simulink model "alimentatorer"  (Simulink 10.0)
settings: Solver=ode15s  StartTime=0.0  StopTime=.5  FixedStep=1e-4  MaxStep=1e-3  RelTol=1e-6  AbsTol=1e-6  EnableMultiTasking=on
settings Model: Creator=prof. G. Celentano  LastModifiedBy=giuseppericcio  ExtModeTrigMode=oneshot  ExtModeArmWhenConnect=off
settings Model: LogicAnalyzerGraphicalSettings=|
  | {
  |   "cursors" : {
  |     "activeCursor" : 0,
  |     "lockedCursors" : [
  | 
  |     ],
  |     "startingCursor" : 0,
  |     "times" : [
  |       0.006
  |     ]
  |   },
  |   "global" : {
  |   },
  |   "panels" : [
  |     {
  |       "height" : 100,
  |       "startingTrace" : 0,
  |       "traces" : [
  | 
  |       ],
  |       "yOffset" : 0
  |     }
  |   ],
  |   "timeAxis" : {
  |     "pixelsPerSecond" : 104998.22050048786
  |   },
  |   "trigger" : {
  |     "enabled" : false,
  |     "mode" : "once",
  |     "samples" : 200,
  |     "signals" : {
  |     },
  |     "stages" : [
  |       {
  |         "conditions" : [
  | 
  |         ],
  |         "operator" : "AND"
  |       }
  |     ]
  |   }
  | }
settings SolverCC: AutoScaleAbsTol=off
settings DataIOCC: SignalLoggingName=sigsOut
settings OptimizationCC: BooleanDataType=off  ExpressionDepthLimit=2147483647
settings DebuggingCC: SaveWithParameterizedLinksMsg=none  SignalResolutionControl=TryResolveAllWithWarning  MultiTaskDSMMsg=warning  MultiTaskCondExecSysMsg=none  FcnCallInpInsideContextMsg=warning  StateNameClashWarn=warning
settings HardwareCC: TargetUnknown=on

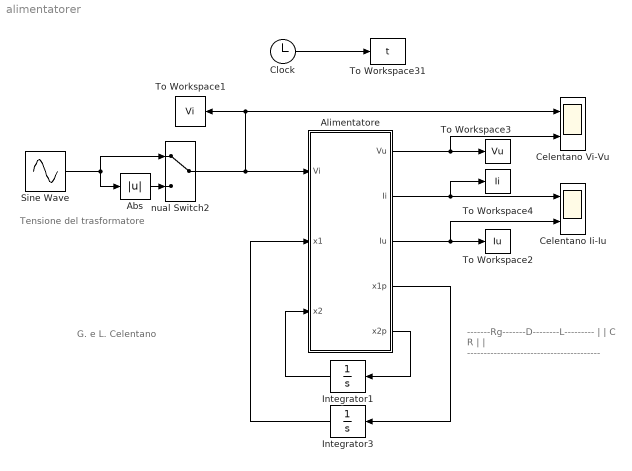
== system alimentatorer ==
  note: Tensione del
      | trasformatore
  note: -------Rg-------D--------L---------
      |                         |         |
      |                         C        R
      |                         |         |
      | ----------------------------------------
  note: G. e L. Celentano
  Abs : Abs  SaturateOnIntegerOverflow=on
  Alimentatore : Subsystem  mask(Alimentatore){Rg=.5, L=5e-1, C=1e-2, R=10}
      mask prompts: Rg "Resistenza del generatore"; L "Induttanza del  filtro"; C "Capacità del filtro"; R "Resistenza di carico"
      mask help: Modello dell'alimentatore
  Celentano Ii-Iu : Scope  NumInputPorts=2
  Celentano Vi-Vu : Scope  NumInputPorts=2
  Clock : Clock
  Integrator1 : Integrator
  Integrator3 : Integrator
  Sine Wave : Sin  Amplitude=10  Frequency=pi*50  SampleTime=0
  To Workspace1 : ToWorkspace  VariableName=Vi  SampleTime=-1
  To Workspace2 : ToWorkspace  VariableName=Iu  SampleTime=-1
  To Workspace3 : ToWorkspace  VariableName=Vu  SampleTime=-1
  To Workspace31 : ToWorkspace  VariableName=t  SampleTime=-1
  To Workspace4 : ToWorkspace  VariableName=Ii  SampleTime=-1
  nual Switch2 : ManualSwitch
  wires:
  Clock/1 -> To Workspace31/1
  Alimentatore/4(x1p) -> Integrator3/1
  Alimentatore/1(Vu) -> Celentano Vi-Vu/2, To Workspace3/1
  Alimentatore/3(Iu) -> To Workspace2/1, Celentano Ii-Iu/2
  Alimentatore/2(Ii) -> Celentano Ii-Iu/1, To Workspace4/1
  Integrator3/1 -> Alimentatore/2(x1)
  Alimentatore/5(x2p) -> Integrator1/1
  Integrator1/1 -> Alimentatore/3(x2)
  Abs/1 -> nual Switch2/2
  Sine Wave/1 -> Abs/1, nual Switch2/1
  nual Switch2/1 -> Alimentatore/1(Vi), To Workspace1/1, Celentano Vi-Vu/1

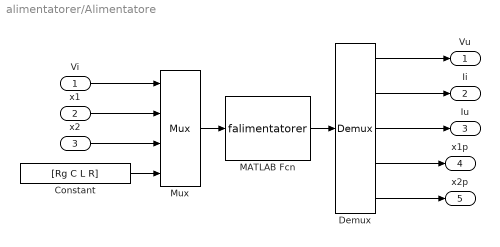
== system alimentatorer/Alimentatore ==
  Vi : Inport
  x1 : Inport  Port=2
  x2 : Inport  Port=3
  Constant : Constant  Value=[Rg C L R]
  Demux : Demux  Outputs=5
  MATLAB Fcn : MATLABFcn  MATLABFcn=falimentatorer  OutputDimensions=5
  Mux : Mux  Inputs=[1 1 1 4]
  Vu : Outport  InitialOutput=0
  Ii : Outport  Port=2  InitialOutput=0
  Iu : Outport  Port=3  InitialOutput=0
  x1p : Outport  Port=4  InitialOutput=0
  x2p : Outport  Port=5  InitialOutput=0
  wires:
  Demux/4 -> x1p/1
  Demux/3 -> Iu/1
  Demux/2 -> Ii/1
  Demux/1 -> Vu/1
  Vi/1 -> Mux/1
  MATLAB Fcn/1 -> Demux/1
  Mux/1 -> MATLAB Fcn/1
  x1/1 -> Mux/2
  Constant/1 -> Mux/4
  x2/1 -> Mux/3
  Demux/5 -> x2p/1
